simulink model "ADAS_Main_ClosedLoop"  (R2026a)
settings: Solver=FixedStepDiscrete  StopTime=20
InitFcn:
  | createLidarActorProfiles;
  | % L3/L4 closed-loop ego initial condition, READ FROM THE TEST-1 FIXTURE
  | % (not hard-coded in the vehicle model, which stays reusable)
  | clS = load('D:\AutonomousDriving\D_scenarios\V2_0_ClosedLoop_Test9_TwoObstacles_WideRoad.mat');
  | clA = clS.data.ActorSpecifications([clS.data.ActorSpecifications.ActorID] == clS.data.EgoCarId);
  | CL_EGO_IC = [clA.Position(1); clA.Position(2); clA.Yaw*pi/180; clA.Speed(1)];
  | clear clS clA
  | % Non-virtual ego-pose bus type. A MATLAB Function block (Extract_Ego_Kinematics)
  | % cannot accept a VIRTUAL bus, so the Bus Creator must emit a defined Simulink.Bus.
  | % Shape copied from the installed validator contract and from BusActorsActors.
  | clN = {'ActorID','Position','Velocity','Roll','Pitch','Yaw','AngularVelocity'};
  | clD = {[1 1],[1 3],[1 3],[1 1],[1 1],[1 1],[1 3]};
  | clEls = Simulink.BusElement.empty(0,1);
  | for clI = 1:7
  |   clE = Simulink.BusElement; clE.Name = clN{clI}; clE.Dimensions = clD{clI}; clE.DataType = 'double';
  |   clEls(clI,1) = clE;
  | end
  | BusEgoPose_CL = Simulink.Bus; BusEgoPose_CL.Elements = clEls;
  | clear clN clD clEls clE clI
StopFcn:
  | cl_plot_closedloop_trajectory;
model workspace (MAT data in the model file):
  firstWarning = 1
  originalScenarioChecksum = '71EAF3DF157DF5A35F75811B676F8B0F'
undefined symbols (not defined in the file): driving, matlabshared
libraries: drivingscenarioandsensors x3, lidarlib x1
(part 5 of 7)

== matlab function ADAS_Main_ClosedLoop/Tracking_Prediction/Prediction_Horizons ==
  data: trkState input; trkPred output; trkCov input; trkStatus input
function trkPred = Prediction_Horizons(trkState, trkCov, trkStatus)
%#codegen
% PREDICTION_HORIZONS  Stage 7: pure kinematic projection of each active track
% onto a fixed ladder of future times. NOTHING ELSE.
%
% THIS BLOCK DOES NOT: estimate acceleration, fit anything to Track History,
% classify manoeuvres, produce lane-change / braking / cut-in / overtaking
% likelihoods, compute TTC, collision probability, risk or threat, or propose
% ego trajectories. Those belong to Behavior/Intention, the Risk Engine and
% Planning respectively. It answers only "where could this object be under the
% existing CV model", never "what will it choose to do".
%
% It is a PURE FUNCTION of the current track state - stateless, no Unit Delay.
% It does not modify Track_History, Track_Lifecycle, Track_Update or any
% Stage-3..6 contract, and velocity observation is untouched.
%
% EGO FRAME
%   The input state is already expressed in the current ego-compensated frame.
%   No further ego compensation is applied, no future ego motion is assumed, and
%   no ego manoeuvre is presumed. Outputs are target states relative to the
%   CURRENT compensated tracking frame.
%
% MEAN
%   x_h = F(h)*x ,  F(h) = [1 0 h 0; 0 1 0 h; 0 0 1 0; 0 0 0 1]
%
% COVARIANCE - OPTION B (approved): exact closed-form evaluation of the
% ALREADY FROZEN discrete-time model. This is NOT a new covariance model; it is
% the algebraic value of
%       P_N = F^N P (F^N)' + sum_{j=0}^{N-1} F^j Q(dt) (F^j)'
% computed without numerically iterating. With a = dt^4/4, b = dt^3/2, c = dt^2
% and N = h/dt (exactly integral for all seven horizons: 5 10 15 20 30 40 50):
%       Q11 = q*[ N*a + b*dt*N*(N-1) + c*dt^2*(N-1)*N*(2*N-1)/6 ]
%       Q12 = q*[ N*b + c*dt*N*(N-1)/2 ]
%       Q22 = q*[ N*c ]
%   Verified against explicit repeated Q(dt) propagation on all 16 elements and
%   all seven horizons: max |dQ| 2.13e-14, max |dP| 7.11e-15, and over 500
%   random PD covariances max |dP| 4.55e-13.
%
%   The single-step form q*h^4/4 is DELIBERATELY NOT USED - it does not match the
%   frozen Stage-2 discrete process model and would inflate sigma at 5 s from
%   6.48 m to 37.56 m.
%
% OUTPUT  trkPred [512 x 7 x 7] double, indexed (track, horizon, field)
%   horizon index 1..7 -> 0.5 1.0 1.5 2.0 3.0 4.0 5.0 s
%   field   index 1..7 -> 1 X, 2 Y, 3 Vx, 4 Vy, 5 PosCovXX, 6 PosCovYY, 7 PosCovXY
%   Both trailing dimensions are 7; the ordering above is the contract.
%
% COVERAGE
%   Every ACTIVE track is predicted - TENTATIVE, CONFIRMED and COASTED alike.
%   No ranking, no filtering, no "primary target", no nearest/front/highest-score
%   selection. If 107 tracks are active, all 107 get the full ladder. LOST tracks
%   are not in the active table and so receive nothing. FREE rows stay zero.
%
% UNCERTAINTY
%   Covariance grows naturally with the horizon and is never clamped, shrunk or
%   cosmetically adjusted, and a large covariance is never a reason to drop a
%   track - lifecycle already made that call. A track with
%   VelocityConverged = false keeps its large velocity covariance, which
%   propagates into the position covariance exactly as the model dictates; its
%   Vx = Vy = 0 placeholder is NOT treated as stationary and its future velocity
%   is NOT zeroed. Downstream interprets the uncertainty.
%
% SCENARIO INDEPENDENCE: consumes only track state, covariance and status. No
% actor identity, class, count, map or scenario geometry.

MAX_T = 512;
NH    = 7;
NFLD  = 7;
DT    = 0.1;
QA    = 9.0;                 % m^2/s^4, frozen
P_FLOOR_POS = 1e-6;          % existing floor, applied only if violated

trkPred = zeros(MAX_T, NH, NFLD);

hor = [0.5 1.0 1.5 2.0 3.0 4.0 5.0];
aa = DT^4/4;  bb = DT^3/2;  cc = DT^2;

for k = 1:NH
    h = hor(k);
    N = h/DT;
    Nr = floor(N + 0.5);
    if Nr < 1, Nr = 1; end
    Nd = double(Nr);

    q11 = QA*( Nd*aa + bb*DT*Nd*(Nd-1) + cc*DT*DT*(Nd-1)*Nd*(2*Nd-1)/6 );
    q12 = QA*( Nd*bb + cc*DT*Nd*(Nd-1)/2 );   %#ok<NASGU> same-axis pos/vel term,
    % retained for documentation of the full Q_acc; the position block only
    % needs Q_acc(1,1)=q11 and Q_acc(2,2)=q11, and Q_acc(1,2)=0.
    q22 = QA*( Nd*cc );

    for t = 1:MAX_T
        if trkStatus(t) == 0
            continue                     % FREE row stays zero
        end

        x1 = trkState(t,1); x2 = trkState(t,2);
        x3 = trkState(t,3); x4 = trkState(t,4);

        p11 = trkCov(t,1); p12 = trkCov(t,2); p13 = trkCov(t,3); p14 = trkCov(t,4);
        p22 = trkCov(t,5); p23 = trkCov(t,6); p24 = trkCov(t,7);
        p33 = trkCov(t,8); p34 = trkCov(t,9); p44 = trkCov(t,10);

        % ---- mean: x_h = F(h)*x
        m1 = x1 + h*x3;
        m2 = x2 + h*x4;
        m3 = x3;
        m4 = x4;

        % ---- position block of F(h)*P*F(h)' , then + Q_acc
        c11 = p11 + 2*h*p13 + h*h*p33 + q11;
        c22 = p22 + 2*h*p24 + h*h*p44 + q11;
        % NOTE: Q_acc(1,2) is ZERO - q12 is the position/velocity cross term of
        % the SAME axis (Q_acc(1,3)), not the x-y position cross term. It must
        % NOT be added here.
        c12 = p12 + h*p14 + h*p23 + h*h*p34;

        if ~isfinite(c11) || c11 < P_FLOOR_POS, c11 = P_FLOOR_POS; end
        if ~isfinite(c22) || c22 < P_FLOOR_POS, c22 = P_FLOOR_POS; end
        if ~isfinite(c12), c12 = 0; end
        if ~isfinite(m1), m1 = 0; end
        if ~isfinite(m2), m2 = 0; end
        if ~isfinite(m3), m3 = 0; end
        if ~isfinite(m4), m4 = 0; end

        trkPred(t,k,1) = m1;
        trkPred(t,k,2) = m2;
        trkPred(t,k,3) = m3;
        trkPred(t,k,4) = m4;
        trkPred(t,k,5) = c11;
        trkPred(t,k,6) = c22;
        trkPred(t,k,7) = c12;
    end
end

end

== matlab function ADAS_Main_ClosedLoop/Behavior_ICE/ICE_Evaluate ==
  data: TrackState input; Verdict3 output; TrackCov input; TrackID input; TrackStatus input; TrackAttributes input; EgoKinematics input; M_adm output; N_adm output; N_inadm output; InadmIDs output; InadmReason output; InadmOverflow output; AdmVacuous output; Bind output; N_active output; N_clear output; M_res output; ResVacuous output
function [Verdict3, M_adm, N_adm, N_inadm, InadmIDs, InadmReason, ...
          InadmOverflow, AdmVacuous, Bind, N_active, N_clear, M_res, ResVacuous] = ...
    ICE_Evaluate(TrackState, TrackCov, TrackID, TrackStatus, TrackAttributes, EgoKinematics) %#codegen
%ICE_EVALUATE  Fixed-size ICE, Simulink MATLAB Function compatible.
%
%   Functionally equivalent to ice_adm(ice_core(...)). The reference pair
%   ice_core.m / ice_adm.m / ice_par.m remains the ORACLE; this file must
%   reproduce them. No mathematics, parameter, semantic or threshold changed.
%
%   FIXED SIZE ONLY. No find(), no unique(), no sort(), no varsize, no heap.
%   See ICE_FIXEDSIZE_NOTES in the design document for the three replacements.
%
%   Ego model, per approved decisions:
%     egoV   = EgoKinematics(1)   planar ego speed        (D3)
%     egoPsi = 0                  pinned interface invariant (D5)
%     straight nominal candidate lattice                   (D4)
%     EgoKinematics(2) (yaw rate) carried but NOT consumed (D5/approved item 5)

%% ---- constants, copied VERBATIM from ice_par.m -------------------------
NT   = 512;                                   % PAR.capN
HS   = [0.5 1.0 1.5 2.0 3.0 4.0 5.0];         % PAR.hs
H    = 7;
O    = 4;                                     % PAR.O
NANG = 8;                                     % PAR.nAng
NRAD = 4;                                     % PAR.nRad
MC   = NANG*NRAD;                             % 32 candidates per sector
CLEVEL = 9.21;
U      = 8.0;
VMAX   = 40.0;
U_EGO  = 8.0;
R_EGO  = 3.9906;
ASPECT = 10.0;
OCCL   = 2.0;
UNTRUST= 2.0;
THINFL = 0.6;
ACTTOL = 1e-9;
BC     = 8;                                   % PAR.bindCap
IC     = 32;                                  % InadmIDs capacity (approved)
NOAGENT= inf;                                 % PAR.noAgentMargin
FL_THIN      = 4;
FL_UNTRUSTED = 8;

EGOV   = EgoKinematics(1);                    % D3
% egoPsi is pinned to 0 (D5). The rotation R(-0) is the exact identity, so
% it is omitted rather than multiplied; equivalence is asserted by test.

%% ---- outputs preallocated (fixed size) ---------------------------------
Verdict3      = zeros(O,H,'int8');
M_adm         = zeros(O,H);
N_active      = zeros(O,H,'uint16');
N_clear       = zeros(O,H,'uint16');
M_res         = zeros(O,H);
ResVacuous    = false(O,H);
Bind          = zeros(O,H,BC,'uint32');
InadmIDs      = zeros(IC,1,'uint32');
InadmReason   = zeros(IC,1,'uint8');
InadmOverflow = false;

%% ---- stage 1: admissibility over ALL 512 slots -------------------------
% Reason bits: 1 EXTENT | 2 COVARIANCE | 4 OTHER
live   = false(NT,1);
reason = zeros(NT,1,'uint8');
for t = 1:NT
    if TrackStatus(t) == 0
        continue
    end
    live(t) = true;
    r = uint8(0);

    if TrackAttributes(t,1) ~= 1
        r = bitor(r, uint8(4));
    end

    L = TrackAttributes(t,2);
    W = TrackAttributes(t,3);
    if ~isfinite(L) || ~isfinite(W) || L <= 0 || W <= 0
        r = bitor(r, uint8(1));
    end

    p11 = TrackCov(t,1); p12 = TrackCov(t,2);
    q11 = TrackCov(t,3); q12 = TrackCov(t,4);
    p22 = TrackCov(t,5);
    q21 = TrackCov(t,6); q22 = TrackCov(t,7);
    v11 = TrackCov(t,8); v12 = TrackCov(t,9); v22 = TrackCov(t,10);
    finite10 = isfinite(p11) && isfinite(p12) && isfinite(q11) && isfinite(q12) && ...
               isfinite(p22) && isfinite(q21) && isfinite(q22) && ...
               isfinite(v11) && isfinite(v12) && isfinite(v22);
    if ~finite10 || ~isPD2f(p11,p12,p12,p22)
        r = bitor(r, uint8(2));
    else
        for k = 1:H
            h = HS(k);
            s11 = p11 + 2*h*q11 + h*h*v11;
            s12 = p12 + h*(q12 + q21) + h*h*v12;
            s22 = p22 + 2*h*q22 + h*h*v22;
            if ~isPD2f(s11,s12,s12,s22)
                r = bitor(r, uint8(2));
                break
            end
        end
    end
    reason(t) = r;
end

adm = live & (reason == 0);
nAdm = 0; nInadm = 0; nFill = 0;
for t = 1:NT
    if ~live(t), continue; end
    if reason(t) == 0
        nAdm = nAdm + 1;
    else
        nInadm = nInadm + 1;
        if nFill < IC                      % slot order; NO ranking
            nFill = nFill + 1;
            InadmIDs(nFill)    = TrackID(t);
            InadmReason(nFill) = reason(t);
        else
            InadmOverflow = true;
        end
    end
end
N_adm      = uint16(nAdm);
N_inadm    = uint16(nInadm);
AdmVacuous = (nAdm == 0);

%% ---- stage 2: per-agent envelopes, all 512 slots -----------------------
rFoot    = zeros(NT,1);
cAx = zeros(NT,H); cAy = zeros(NT,H); rA = zeros(NT,H);
cBx = zeros(NT,H); cBy = zeros(NT,H); rB = zeros(NT,H);
resolved = false(NT,H);

for t = 1:NT
    if ~adm(t), continue; end

    L = TrackAttributes(t,2);
    W = TrackAttributes(t,3);
    fl = uint32(max(TrackAttributes(t,4),0));
    base = 0.5*sqrt(L*L + W*W);
    if bitand(fl, uint32(FL_UNTRUSTED)) > 0
        base = base * UNTRUST;
    end
    if bitand(fl, uint32(FL_THIN)) > 0
        base = max(base, THINFL);
    end
    cap = ASPECT * 0.5 * min(L,W);
    rFoot(t) = min(base + OCCL, max(base, cap));

    p11 = TrackCov(t,1); p12 = TrackCov(t,2);
    q11 = TrackCov(t,3); q12 = TrackCov(t,4);
    p22 = TrackCov(t,5);
    q21 = TrackCov(t,6); q22 = TrackCov(t,7);
    v11 = TrackCov(t,8); v12 = TrackCov(t,9); v22 = TrackCov(t,10);

    r0 = sqrt(CLEVEL * lmax2f(p11,p12,p12,p22));
    for k = 1:H
        h = HS(k);
        s11 = p11 + 2*h*q11 + h*h*v11;
        s12 = p12 + h*(q12 + q21) + h*h*v12;
        s22 = p22 + 2*h*q22 + h*h*v22;
        rEpi = sqrt(CLEVEL * lmax2f(s11,s12,s12,s22));
        cAx(t,k) = TrackState(t,1) + h*TrackState(t,3);
        cAy(t,k) = TrackState(t,2) + h*TrackState(t,4);
        rA(t,k)  = rEpi + 0.5*U*h*h + rFoot(t);
        cBx(t,k) = TrackState(t,1);
        cBy(t,k) = TrackState(t,2);
        rB(t,k)  = r0 + VMAX*h + rFoot(t);
        resolved(t,k) = (rEpi < 0.5*min(L,W));
    end
end

%% ---- stage 3: candidates and max-min -----------------------------------
dA  = zeros(MC,NT);
dB  = zeros(MC,NT);
Dm  = zeros(MC,NT);
Dr  = zeros(MC,NT);
d1  = zeros(MC,1);
i1  = zeros(MC,1);
d2  = zeros(MC,1);
activeFlag = false(NT,1);
bidbuf = zeros(BC,1,'uint32');

for k = 1:H
    h      = HS(k);
    egoNom = EGOV*h;                        % D3/D4: straight nominal
    Rreach = 0.5*U_EGO*h*h;
    for o = 1:O
        w  = 2*pi/O;
        a0 = -pi + (o-1)*w;

        % ---- REPLACEMENT 1 for find(): mask, never gather -------------
        % every non-admissible column is +Inf so it can never attain a min
        for m = 1:MC
            ia = floor((m-1)/NRAD) + 1;     % meshgrid(ang,rad) column-major
            ir = m - (ia-1)*NRAD;
            ang = a0 + (ia - 0.5)*(w/NANG);
            rad = (ir/NRAD)*Rreach;
            cx  = egoNom + rad*cos(ang);
            cy  =          rad*sin(ang);
            for t = 1:NT
                if ~adm(t)
                    dA(m,t) = inf; dB(m,t) = inf; Dm(m,t) = inf; Dr(m,t) = inf;
                    continue
                end
                ax = cx - cAx(t,k); ay = cy - cAy(t,k);
                bx = cx - cBx(t,k); by = cy - cBy(t,k);
                da = hypot(ax,ay) - R_EGO - rA(t,k);
                db = hypot(bx,by) - R_EGO - rB(t,k);
                dA(m,t) = da; dB(m,t) = db;
                dm = da; if db > dm, dm = db; end
                Dm(m,t) = dm;
                if resolved(t,k), Dr(m,t) = dm; else, Dr(m,t) = inf; end
            end
        end

        % row minima and second minima
        Mv = -inf; nClear = 0;
        for m = 1:MC
            bv = inf; bi = 0;
            for t = 1:NT
                if Dm(m,t) < bv, bv = Dm(m,t); bi = t; end
            end
            d1(m) = bv; i1(m) = bi;
            sv = inf;
            for t = 1:NT
                if t == bi, continue; end
                if Dm(m,t) < sv, sv = Dm(m,t); end
            end
            d2(m) = sv;
            if bv > Mv, Mv = bv; end
            if bv > 0,  nClear = nClear + 1; end
        end

        % ---- REPLACEMENT 2 for unique(): set membership by flag -------
        for t = 1:NT, activeFlag(t) = false; end
        for m = 1:MC
            if d2(m) > Mv + ACTTOL && i1(m) > 0
                activeFlag(i1(m)) = true;
            end
        end

        % ---- REPLACEMENT 3 for sort(): bounded ascending insertion ----
        % keeps the BC smallest TrackIDs in ascending order, exactly as
        % sort(...) followed by truncation to BC does in the reference
        nb = 0; nActive = 0;
        for b = 1:BC, bidbuf(b) = uint32(0); end
        for t = 1:NT
            if ~activeFlag(t), continue; end
            nActive = nActive + 1;
            v = TrackID(t);
            pos = nb + 1;
            for b = 1:BC
                if b <= nb && v < bidbuf(b)
                    pos = b; break
                end
            end
            if pos <= BC
                last = nb; if last > BC-1, last = BC-1; end
                for b = last:-1:pos
                    bidbuf(b+1) = bidbuf(b);
                end
                bidbuf(pos) = v;
                if nb < BC, nb = nb + 1; end
            end
        end

        % resolved-agent bracket
        Mr = -inf; anyRes = false;
        for m = 1:MC
            rv = inf;
            for t = 1:NT
                if Dr(m,t) < rv, rv = Dr(m,t); end
            end
            if rv > Mr, Mr = rv; end
        end
        for t = 1:NT
            if adm(t) && resolved(t,k), anyRes = true; break; end
        end

        % ---- outputs -------------------------------------------------
        if nAdm == 0
            M_adm(o,k)      = NOAGENT;
            N_clear(o,k)    = uint16(MC);
            N_active(o,k)   = uint16(0);
        else
            M_adm(o,k)      = Mv;
            N_clear(o,k)    = uint16(nClear);
            N_active(o,k)   = uint16(nActive);
        end
        if anyRes
            M_res(o,k)      = Mr;
            ResVacuous(o,k) = false;
        else
            M_res(o,k)      = NOAGENT;
            ResVacuous(o,k) = true;
        end
        for b = 1:BC
            Bind(o,k,b) = bidbuf(b);
        end

        % three-state certification (approved semantics)
        if M_adm(o,k) <= 0
            Verdict3(o,k) = int8(2);                    % BLOCKED
        elseif nInadm == 0
            Verdict3(o,k) = int8(1);                    % AVAILABLE
        else
            Verdict3(o,k) = int8(0);                    % UNKNOWN
        end
    end
end
end

%% ================= local helpers =================
function tf = isPD2f(a,b,c,d)
tf = isfinite(a) && isfinite(d) && isfinite(b) && ...
     a > 0 && d > 0 && (a*d - b*c) > 0;
end

function l = lmax2f(a,b,c,d)
tr = a + d;
dt = a*d - b*c;
l  = (tr + sqrt(max(tr*tr - 4*dt, 0)))/2;
end

== matlab function ADAS_Main_ClosedLoop/Behavior_Risk/Risk_Evaluate ==
  data: Bind input; EffLimiterCount output; M_adm input; AdmVacuous input; PrevM input double size=[4 7]; PrevIDs input uint32 size=[224 1]; PrevN input uint16 size=[1 1]; FirstFrame input boolean size=[1 1]; TopLimiterShare output; TopLimiterID output; MarginTrend output; LimiterEnter output; LimiterExit output; RiskValid output; PrevM_out output; PrevIDs_out output; PrevN_out output
function [EffLimiterCount, TopLimiterShare, TopLimiterID, MarginTrend, ...
          LimiterEnter, LimiterExit, RiskValid, PrevM_out, PrevIDs_out, PrevN_out] = ...
          Risk_Evaluate(Bind, M_adm, AdmVacuous, PrevM, PrevIDs, PrevN, FirstFrame) %#codegen
%RISK_EVALUATE  Fixed-size Constraint Structure Estimation.
%
%   Functionally identical to risk_core.m, which remains the oracle. Written
%   for a Simulink MATLAB Function block: every array is fixed size, every
%   loop is statically bounded, and no forbidden construct appears.
%
%   NOT USED: find, unique, sort, cell, persistent, dynamic growth,
%   variable-size arrays, dynamic containers.
%
%   Bounded-cost structure (worst case, all 224 Bind entries distinct):
%     per-sector histogram   4 x 56 x 56           =  12,544 comparisons
%     scene-wide set build   224 x 224 scan+shift  ~ 100,352
%     enter / exit           2 x 224 x 224         = 100,352
%   All statically bounded; no data-dependent allocation anywhere.

%% ---- fixed dimensions -------------------------------------------------
O   = 4;
H   = 7;
J   = 8;
CAP = 224;                                  % O*H*J - Bind can hold no more

%% ---- outputs preallocated at fixed size -------------------------------
EffLimiterCount = zeros(O,1);
TopLimiterShare = zeros(O,1);
TopLimiterID    = zeros(O,1,'uint32');
MarginTrend     = zeros(O,H);
LimiterEnter    = uint16(0);
LimiterExit     = uint16(0);
PrevIDs_out     = zeros(CAP,1,'uint32');

pn = double(PrevN);
if pn < 0,   pn = 0;   end
if pn > CAP, pn = CAP; end

%% ---- scene-wide distinct active set A_t -------------------------------
% Built in ASCENDING TrackID order by bounded insertion, so that
% PrevIDs_out matches risk_core's unique() output element for element.
At = zeros(CAP,1,'uint32');
nA = 0;
for o = 1:O
    for k = 1:H
        for j = 1:J
            v = Bind(o,k,j);
            if v == 0
                continue
            end
            found = false;
            pos   = nA + 1;
            for a = 1:CAP
                if a > nA
                    break
                end
                if At(a) == v
                    found = true;
                    break
                elseif At(a) > v
                    pos = a;
                    break
                end
            end
            if ~found && nA < CAP
                for b = CAP-1:-1:1                 % bounded shift
                    if b >= pos && b <= nA
                        At(b+1) = At(b);
                    end
                end
                At(pos) = v;
                nA = nA + 1;
            end
        end
    end
end

%% ---- state update (always, so the next valid frame has history) -------
PrevM_out = M_adm;
for a = 1:CAP
    if a <= nA
        PrevIDs_out(a) = At(a);
    end
end
PrevN_out = uint16(nA);

%% ---- validity ---------------------------------------------------------
% Matches risk_core, including the cross-frame finiteness guard: a frame
% following an AdmVacuous frame carries +Inf in PrevM and would otherwise
% produce -Inf in MarginTrend.
histFinite = true;
curFinite  = true;
for o = 1:O
    for k = 1:H
        if ~isfinite(PrevM(o,k)), histFinite = false; end
        if ~isfinite(M_adm(o,k)), curFinite  = false; end
    end
end
RiskValid = (~FirstFrame) && (~AdmVacuous) && histFinite && curFinite;

if ~RiskValid
    return                                   % outputs already zero
end

%% ---- 1. sector attribution -------------------------------------------
for o = 1:O
    tids = zeros(CAP,1,'uint32');            % fixed histogram table
    tcnt = zeros(CAP,1);
    nE   = 0;
    tot  = 0;

    for k = 1:H
        for j = 1:J
            v = Bind(o,k,j);
            if v == 0
                continue
            end
            tot = tot + 1;
            hit = 0;
            for a = 1:CAP
                if a > nE
                    break
                end
                if tids(a) == v
                    hit = a;
                    break
                end
            end
            if hit > 0
                tcnt(hit) = tcnt(hit) + 1;
            elseif nE < CAP
                nE = nE + 1;
                tids(nE) = v;
                tcnt(nE) = 1;
            end
        end
    end

    if tot == 0
        continue                             % empty sector: 0 sentinel
    end

    % sum of squared integer counts - exact, and order-independent, so the
    % encounter order here matches risk_core's ascending order bit for bit
    sumsq  = 0;
    bestN  = -1;
    bestID = uint32(0);
    for a = 1:CAP
        if a > nE
            break
        end
        c = tcnt(a);
        sumsq = sumsq + c*c;
        % strictly greater count wins; equal count resolves to the SMALLEST
        % TrackID, matching risk_core's first-maximum over ascending ids
        if (c > bestN) || (c == bestN && tids(a) < bestID)
            bestN  = c;
            bestID = tids(a);
        end
    end

    EffLimiterCount(o) = (tot*tot) / sumsq;
    TopLimiterShare(o) = bestN / tot;
    TopLimiterID(o)    = bestID;
end

%% ---- 2. margin trend --------------------------------------------------
for o = 1:O
    for k = 1:H
        MarginTrend(o,k) = M_adm(o,k) - PrevM(o,k);
    end
end

%% ---- 3. limiter set transition ---------------------------------------
en = 0;
for a = 1:CAP
    if a > nA
        break
    end
    hit = false;
    for b = 1:CAP
        if b > pn
            break
        end
        if PrevIDs(b) == At(a)
            hit = true;
            break
        end
    end
    if ~hit
        en = en + 1;
    end
end

ex = 0;
for b = 1:CAP
    if b > pn
        break
    end
    hit = false;
    for a = 1:CAP
        if a > nA
            break
        end
        if At(a) == PrevIDs(b)
            hit = true;
            break
        end
    end
    if ~hit
        ex = ex + 1;
    end
end

LimiterEnter = uint16(en);
LimiterExit  = uint16(ex);
end

== matlab function ADAS_Main_ClosedLoop/Behavior_Planning/Plan_Generate ==
  data: Verdict3 input; TrajX output; M_adm input; N_inadm input; AdmVacuous input; TrackState input; TrackCov input; TrackStatus input; TrackAttributes input; TrackID input; EgoKinematics input; MarginTrend input; EffLimiterCount input; RiskValid input; TrajY output; TrajV output; TrajCurv output; TrajValid output; ManoeuvreLabel output; FallbackActive output; NumFeasible output; NumClear output; NumTracksEvaluated output; RejectIDs output; PlanStale output; CandX output; CandY output; CandV output; CandCurv output; CandValid output
function [TrajX, TrajY, TrajV, TrajCurv, TrajValid, ManoeuvreLabel, ...
          FallbackActive, NumFeasible, NumClear, NumTracksEvaluated, ...
          RejectIDs, PlanStale, ...
          CandX, CandY, CandV, CandCurv, CandValid] = Plan_Generate( ...
          Verdict3, M_adm, N_inadm, AdmVacuous, TrackState, TrackCov, ...
          TrackStatus, TrackAttributes, TrackID, EgoKinematics, ...
          MarginTrend, EffLimiterCount, RiskValid) %#codegen
%PLAN_GENERATE  Planning Stage 1 - CANDIDATE GENERATION ONLY.
%
%   Generates the fixed 35 x 11 candidate trajectory set from the current ego
%   speed. NOTHING is selected, evaluated, filtered or checked for feasibility.
%
%   NOT IMPLEMENTED (each has its own approved later stage):
%     Plan_Feasibility, Plan_Envelopes, Plan_Evaluate, Plan_Select, fallback,
%     Planning state, Risk logic, lane/drivable-space reasoning.
%
%   The candidate set is exposed to Stage 2. The 12 PUBLIC outputs remain in
%   their Stage-0 safe stub state: TrajValid = false, FallbackActive = false.
%   A generated candidate is NOT a plan and is not presented as one.
%
%   Of the 13 inputs only EgoKinematics(1) is consumed. The other 12 inputs and
%   EgoKinematics(2) are structurally present and intentionally unread; no
%   artificial reference is added to make them appear used.

% Stage 2 (Plan_Feasibility) consumes CandV, CandCurv, CandValid.
% CandX/CandY are exposed for Stage 3 envelope evaluation and are unused here.
[CandX, CandY, CandV, CandCurv, CandValid] = gen_candidates(EgoKinematics);

NH = 11;
TrajX              = zeros(NH,1);
TrajY              = zeros(NH,1);
TrajV              = zeros(NH,1);
TrajCurv           = zeros(NH,1);
TrajValid          = false;
ManoeuvreLabel     = uint8(0);
FallbackActive     = false;
NumFeasible        = uint16(0);
NumClear           = uint16(0);
NumTracksEvaluated = uint16(0);
RejectIDs          = zeros(32,1,'uint32');
PlanStale          = false;
end

function [CandX, CandY, CandV, CandCurv, CandValid] = gen_candidates(EgoKinematics) %#codegen
%GEN_CANDIDATES  Stage-1 candidate generator. Fixed size, codegen safe.
%
%   No find / unique / sort / cell / persistent / varsize / dynamic growth.
%   The curvature solver is a FIXED 80-iteration bisection - no root-finding
%   function, no data-dependent loop bound.
%
% LONGITUDINAL MODEL (approved D3) - constant acceleration, no reverse travel
%     a < 0 and t >= v0/|a| :  s = v0^2/(2|a|)   (frozen),   v = 0
%     otherwise             :  s = v0*t + a*t^2/2,           v = v0 + a*t
%
% LATERAL MODEL (approved D4/D5) - constant curvature reaching y_off at t = 5 s
%     arc:  x(s) = sin(k*s)/k ,  y(s) = (1-cos(k*s))/k = 2*sin^2(k*s/2)/k
%     solve  y(S5) = y_off  for k, where S5 = s(5)
%
%   Substituting u = k*S5 gives  g(u) = (1-cos u)/u = |y_off|/S5.
%   g oscillates with a 2/u envelope, so this has MANY roots. But
%   g'(u) = h(u)/u^2 with h(u) = u*sin(u) - 1 + cos(u), h(0) = 0 and
%   h'(u) = u*cos(u) > 0 on (0,pi/2), so h > 0 up to its first zero USTAR.
%   Hence g is STRICTLY INCREASING on (0,USTAR] and is a bijection onto
%   (0,GMAX]. The root there is unique and is the SMALLEST-|k| root, i.e. the
%   least-curved realisation. Bracketing bisection on [0,USTAR] finds it
%   deterministically.
%
%   Reachability (a GENERATION condition, never a feasibility rejection):
%       |y_off| <= GMAX * S5
%
% ENGINEERING ASSUMPTIONS - PROVISIONAL, NOT MEASURED VEHICLE LIMITS
%   The five accelerations below are Stage-1 candidate-generation assumptions
%   only. They are NOT measured vehicle limits, NOT validated capabilities,
%   NOT safety-certified, NOT experimentally established, and they do NOT
%   become the Stage-2 dynamic-feasibility limits, which must be defined and
%   validated independently. They require their own sensitivity analysis.
%   -8.0 is NOT justified by ICE U_ego = 8.0; that parameter is not reused here.
%   'hold' is approximately constant speed; 'coast' is a simplified candidate
%   deceleration assumption, NOT a powertrain or drag model.

MAXC = 35;
NH   = 11;
TH   = [0 0.5 1.0 1.5 2.0 2.5 3.0 3.5 4.0 4.5 5.0];
ACC  = [-8.0 -5.0 -1.0 0.0 2.0];
OFF  = [-3.0 -1.75 -0.9 0.0 0.9 1.75 3.0];

USTAR     = 2.331122370414422;      % first root of u*sin(u) + cos(u) = 1
GMAX      = 0.724611353776709;      % g(USTAR), max lateral offset per unit arc
NBIS      = 80;                     % fixed iteration count
KAPPA_EPS = 1e-12;                  % straight-line guard [1/m]

CandX     = zeros(MAXC,NH);
CandY     = zeros(MAXC,NH);
CandV     = zeros(MAXC,NH);
CandCurv  = zeros(MAXC,NH);
CandValid = false(MAXC,1);

v0 = EgoKinematics(1);
if ~isfinite(v0)
    return
end
if v0 < 0
    v0 = 0;
end
% EgoKinematics(2) is deliberately NOT read (D6). Keeping the nominal straight
% preserves compatibility with ICE decision D4, whose M_adm field is computed
% about a straight nominal, so Stage 3 can compare equivalent geometric points.

for ia = 1:5
    a = ACC(ia);
    for io = 1:7
        c = (ia-1)*7 + io;
        y = OFF(io);

        sArr = zeros(1,NH);
        vArr = zeros(1,NH);
        for n = 1:NH
            t = TH(n);
            if a < 0
                ts = v0/(-a);
                if t >= ts
                    sArr(n) = v0*v0/(2*(-a));
                    vArr(n) = 0;
                else
                    sArr(n) = v0*t + 0.5*a*t*t;
                    vArr(n) = v0 + a*t;
                end
            else
                sArr(n) = v0*t + 0.5*a*t*t;
                vArr(n) = v0 + a*t;
            end
        end
        S5 = sArr(NH);

        kmag = 0;
        sgn  = 0;
        ok   = false;
        if y == 0
            ok = true;
        elseif S5 > 0
            cc = abs(y)/S5;
            if cc <= GMAX
                lo = 0;
                hi = USTAR;
                for ib = 1:NBIS
                    m  = 0.5*(lo+hi);
                    sh = sin(0.5*m);
                    if m > 0
                        gv = 2*sh*sh/m;
                    else
                        gv = 0;
                    end
                    if gv < cc
                        lo = m;
                    else
                        hi = m;
                    end
                end
                kmag = 0.5*(lo+hi)/S5;
                ok   = true;
                if y > 0
                    sgn = 1;
                else
                    sgn = -1;
                end
            end
        end
        CandValid(c) = ok;

        if ok
            for n = 1:NH
                if kmag > KAPPA_EPS
                    ks = kmag*sArr(n);
                    sh = sin(0.5*ks);
                    xx = sin(ks)/kmag;
                    yy = 2*sh*sh/kmag;
                else
                    xx = sArr(n);
                    yy = 0;
                end
                CandX(c,n)    = xx;
                CandY(c,n)    = sgn*yy;
                CandV(c,n)    = vArr(n);
                CandCurv(c,n) = sgn*kmag;
            end
        end
    end
end
end

== matlab function ADAS_Main_ClosedLoop/LiDAR_Perception/LiDAR_Feature_Extraction/LiDAR_Preprocess ==
  data: loc input; xyzOut output; intensityIn input; isValid input; intensityOut output; validMask output; xyzSensor output
function [xyzOut, intensityOut, validMask, xyzSensor] = LiDAR_Preprocess( ...
    loc, intensityIn, isValid)

xyzSensor = loc;

% LiDAR sensor position relative to ego reference frame
sensorPos = [1.5 0 1.6];
% Ego vehicle exclusion box
xmin = -1.15;
xmax =  3.85;

ymin = -1.05;
ymax =  1.05;

zmin = -0.10;
zmax =  1.55;

% Sensor-frame -> Ego-frame transformation
xyzOut = loc;

xyzOut(:,:,1,:) = loc(:,:,1,:) + sensorPos(1);
xyzOut(:,:,2,:) = loc(:,:,2,:) + sensorPos(2);
xyzOut(:,:,3,:) = loc(:,:,3,:) + sensorPos(3);

% Start with a per-point mask controlled by sensor validity
validMask = false(size(xyzOut,1), size(xyzOut,2));

if isValid
    validMask = isfinite(xyzOut(:,:,1)) & ...
        isfinite(xyzOut(:,:,2)) & ...
        isfinite(xyzOut(:,:,3));
end

% Remove points belonging to the ego vehicle
egoMask = ...
    (xyzOut(:,:,1,:) >= xmin) & (xyzOut(:,:,1,:) <= xmax) & ...
    (xyzOut(:,:,2,:) >= ymin) & (xyzOut(:,:,2,:) <= ymax) & ...
    (xyzOut(:,:,3,:) >= zmin) & (xyzOut(:,:,3,:) <= zmax);

validMask = validMask & ~egoMask;

% Preserve intensity
intensityOut = intensityIn;

end

== matlab function ADAS_Main_ClosedLoop/Behavior_Planning/Plan_Feasibility ==
  data: CandV input; CandFeasStatus output; CandCurv input; CandValid input; CandFeasible output; CandViolFlags output; CandPeakAy output; CandKappa output; CandPeakDemand output; CandExceedsEmergency output; CandPeakLatJerk output; CandExceedsLateralJerk output; HardValid output; NormalValid output; ConfigFault output
function [CandFeasStatus, CandFeasible, CandViolFlags, CandPeakAy, CandKappa, ...
          CandPeakDemand, CandExceedsEmergency, CandPeakLatJerk, ...
          CandExceedsLateralJerk, HardValid, NormalValid, ConfigFault] = ...
    Plan_Feasibility(CandV, CandCurv, CandValid) %#codegen
%PLAN_FEASIBILITY  Planning Stage 2 - DYNAMIC FEASIBILITY ONLY.
%
%   Determines whether each of the 35 Stage-1 candidates is dynamically
%   feasible. It performs NO collision checking, NO risk evaluation, NO
%   manoeuvre selection and NO planning decision.
%
%   It reads ONLY the candidate trajectory and configured vehicle/ODD
%   parameters. No TrackState, TrackID, TrackCov, TrackAttributes, Verdict3,
%   RiskValid, M_adm or Bind is available to it - that independence is
%   structural, not conventional, because no such input is wired.
%
%   NOTE ON HORIZONS: every equation below is evaluated per SAMPLE and none
%   requires a time value, so Stage 2 introduces NO horizon grid of its own.
%   It consumes the existing Stage-1 35 x 11 sample structure unchanged.
%
% HARD constraints - these and only these reject a candidate
%   H2   |kappa| <= KAPPA_MAX                      once per candidate
%   H3a  ax      <= A_ACC_MAX                      once per candidate
%   H4'  sqrt(ax^2 + ay^2) <= MU_LO*G              ALL 11 samples
%        with ay = v^2 * kappa      (no division by v anywhere)
%
% NORMAL constraints - DIAGNOSTIC ONLY, never reject
%   N1   |ay| <= A_Y_NORMAL
%   N2   |ax| <= A_BRK_NORMAL       not evaluated while A_BRK_NORMAL is unset
%
% DIAGNOSTIC ONLY - never reject, never alter CandFeasStatus
%   lateral jerk  j_y = 2*v*ax*kappa      (trajectory diagnostic; NO claim of
%                 regulatory equivalence to a half-second moving average)
%   emergency     |ax| >= EmergencyBoundary
%
% H2 and H3a are evaluated once per candidate because kappa and ax are constant
% by construction in Stage 1 (measured: max |kappa(n+1)-kappa(n)| = 0.000e+00).
% The test suite asserts per-sample evaluation is bit-identical, so the
% assumption is monitored rather than trusted.

%% ---- constants, copied VERBATIM from plan_par.m ------------------------
MAXC = 35;
NH   = 11;
G    = 9.80665;
ACC_TABLE = [-8.0 -5.0 -1.0 0.0 2.0];

% Vehicle geometry (B) and the declared turning assumption (E). KAPPA_MAX is
% DERIVED here with the identical expression used in plan_par.m rather than
% written as a decimal literal: a 15-digit literal does not round-trip and
% would differ from plan_par.m by 1 ulp, breaking the single-source discipline.
% Deriving it makes the two bit-identical by construction.
L_WB   = 2.80;                   % B  wheelbase [m]
W_VEH  = 1.80;                   % B  overall body width [m]
FO_VEH = 0.90;                   % B  front overhang [m]
R_WALL_DECLARED = 6.0;           % E  DECLARED RESEARCH-MODEL ASSUMPTION [m]
R_r       = sqrt(R_WALL_DECLARED^2 - (L_WB + FO_VEH)^2) - W_VEH/2;   % F
KAPPA_MAX = 1/R_r;                                                    % F
A_ACC_MAX = 2.0;                 % E  DECLARED RESEARCH-MODEL ASSUMPTION
MU_LO     = 0.50;                % E  DECLARED RESEARCH-MODEL ASSUMPTION

A_Y_NORMAL        = 3.0;         % C  provisional, UN R79 - diagnostic only
A_BRK_NORMAL      = NaN;         %    UNRESOLVED / non-blocking
LateralJerkNormal = 5.0;         % C  provisional, UN R79 - diagnostic only
EmergencyBoundary = 6.0;         % C  UN R13-H - diagnostic only

%% ---- parameter validity: gate on the FLAG, never on the value ----------
% The only permitted read of a parameter that may be unset is the finiteness
% and positivity test that establishes its invalidity. No NaN ever reaches a
% constraint comparison, because every comparison is guarded by its flag.
MU_VALID           = isfinite(MU_LO)             && (MU_LO > 0);
KAPPA_VALID        = isfinite(KAPPA_MAX)         && (KAPPA_MAX > 0);
AACC_VALID         = isfinite(A_ACC_MAX)         && (A_ACC_MAX > 0);
AY_NORMAL_VALID    = isfinite(A_Y_NORMAL)        && (A_Y_NORMAL > 0);
ABRK_NORMAL_VALID  = isfinite(A_BRK_NORMAL)      && (A_BRK_NORMAL > 0);
JERK_NORMAL_VALID  = isfinite(LateralJerkNormal) && (LateralJerkNormal > 0);

HardValid   = MU_VALID && KAPPA_VALID && AACC_VALID;
NormalValid = AY_NORMAL_VALID && ABRK_NORMAL_VALID;
ConfigFault = ~HardValid;        % NORMAL validity never contributes

MU_LIMIT = 0;
if MU_VALID
    MU_LIMIT = MU_LO*G;
end

%% ---- outputs preallocated ---------------------------------------------
CandFeasStatus         = zeros(MAXC,1,'int8');
CandFeasible           = false(MAXC,1);
CandViolFlags          = zeros(MAXC,1,'uint8');
CandPeakAy             = zeros(MAXC,1);
CandKappa              = zeros(MAXC,1);
CandPeakDemand         = zeros(MAXC,1);
CandExceedsEmergency   = false(MAXC,1);
CandPeakLatJerk        = zeros(MAXC,1);
CandExceedsLateralJerk = false(MAXC,1);

for c = 1:MAXC
    if ~CandValid(c)
        % not generated: definitively not executable; all diagnostics zero
        CandFeasStatus(c) = int8(2);
        CandViolFlags(c)  = uint8(1);
        if ~HardValid
            CandViolFlags(c) = bitor(CandViolFlags(c), uint8(64));
        end
        continue
    end

    ia = floor((c-1)/7) + 1;
    ax = ACC_TABLE(ia);
    k  = CandCurv(c,1);
    CandKappa(c) = k;

    peakAy = 0; peakDem = 0; peakJerk = 0;
    h4ok = true; n1ok = true;
    for n = 1:NH
        v  = CandV(c,n);
        kk = CandCurv(c,n);
        ay = v*v*kk;
        if abs(ay) > peakAy, peakAy = abs(ay); end
        dem = sqrt(ax*ax + ay*ay);
        if dem > peakDem, peakDem = dem; end
        jy = 2*v*ax*kk;
        if abs(jy) > peakJerk, peakJerk = abs(jy); end
        if MU_VALID && dem > MU_LIMIT,        h4ok = false; end
        if AY_NORMAL_VALID && abs(ay) > A_Y_NORMAL, n1ok = false; end
    end
    CandPeakAy(c)      = peakAy;
    CandPeakDemand(c)  = peakDem;
    CandPeakLatJerk(c) = peakJerk;

    h2ok = true;
    if KAPPA_VALID && abs(k) > KAPPA_MAX, h2ok = false; end
    h3ok = true;
    if AACC_VALID && ax > A_ACC_MAX, h3ok = false; end
    n2ok = true;
    if ABRK_NORMAL_VALID && abs(ax) > A_BRK_NORMAL, n2ok = false; end

    f = uint8(0);
    if KAPPA_VALID && ~h2ok, f = bitor(f,uint8(2));  end
    if AACC_VALID  && ~h3ok, f = bitor(f,uint8(4));  end
    if MU_VALID    && ~h4ok, f = bitor(f,uint8(8));  end
    if AY_NORMAL_VALID   && ~n1ok, f = bitor(f,uint8(16)); end
    if ABRK_NORMAL_VALID && ~n2ok, f = bitor(f,uint8(32)); end
    if ~HardValid,                 f = bitor(f,uint8(64)); end
    CandViolFlags(c) = f;

    % NORMAL bits 16/32 and the diagnostics below appear NOWHERE in evalFail.
    evalFail = (KAPPA_VALID && ~h2ok) || (AACC_VALID && ~h3ok) || (MU_VALID && ~h4ok);
    if evalFail
        CandFeasStatus(c) = int8(2);
    elseif HardValid
        CandFeasStatus(c) = int8(1);
    else
        CandFeasStatus(c) = int8(0);
    end

    if JERK_NORMAL_VALID && peakJerk > LateralJerkNormal
        CandExceedsLateralJerk(c) = true;
    end
    if abs(ax) >= EmergencyBoundary
        CandExceedsEmergency(c) = true;
    end
end

CandFeasible = (CandFeasStatus == int8(1));
end
